simulink model "drive_cycle"  (R2019b)
settings: Solver=VariableStepAuto  StartTime=0.0  StopTime=1561  RelTol=1e-3
model workspace (MATLAB code in the model file):
  | ms = 135;
  | mf = 5;
  | mr = 10;
  | m = ms + (mf + mr);
  | a = 0.7;
  | b = 0.7;
  | Cd = 0.8;
  | Af = 1;
  | h_cg = 0.5;
  | kf = 10000;
  | kr = 15000;
  | cf = 5000;
  | cr = 5000;
  | I = 500;
  | kt = 175000;
  | GR = 6.5;
  | Pmax = 5500;
  | Tmax = 26;
libraries: autolibshared x4
(part 1 of 3)
settings Model: Creator=Barath Krishna S  LastModifiedBy=Barath Krishna S

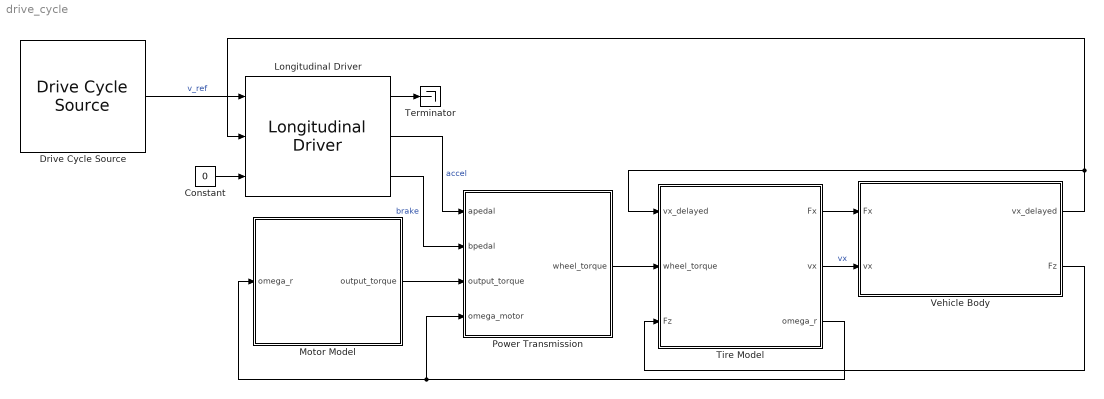
== system drive_cycle ==
  Constant : Constant  Value=0
  Drive Cycle Source : autolibshared/Drive Cycle Source  cycleVar=Workspace variable  wsVar=mycycle  fileVar=cycleFTP75.mat  tfinal="1560.636  seconds"  cycleRepeat=off  outAccPort=off  outGearPort=off  gearList=No gear data  t_wot1=5  xdot_woto=0  xdot_wot1=30  t_wot2=20  xdot_wot2=0  t_wotend=30  srcUnit=m/s  outUnit=m/s  srcAccUnit=m/s/s  outAccUnit=m/s^2  dt=0  aMode=1
      settings: SourceProductName=Powertrain Blockset  SourceProductBaseCode=PW
  Longitudinal Driver : autolibshared/Longitudinal Driver  cntrlType=PI  shftType=None  velUnits=m/s  gearOut=off  Kp=100  Ki=2.5  Kff=.05  Kg=.01  VehVelVec=[0 100]  KffVec=[.1 .1]  KpVec=[10 10]  KiVec=[5 5]  KgVec=[0 0]  m=1500  Kpt=3000  tau=.1  L=2  aR=200  bR=2.5  cR=.5  g=9.81  vnom=100  Kaw=.1  tauerr=.03  tauPt=2  GearInit=0  tShift=.1  pdlVec=[0.1 0.4 0.5 0.9]  upShftTbl=[-1 12.9375 26.4375 39.9375 51.18749999999999 62.4375 72.84375 83.25;-1 16.3125 29.8125 43.3125 54.5624 65.8125 76.78125 87.75;-1 19.6875 33.1875 46.68749999999999 57.9375 69.1875 80.71875 92.25;-1 33 52.5 77.25 100.5 138.75 161.875 185]  dwnShftTbl=[1 9.5625 23.0625 36.5625 47.8125 59.0625 68.90625 78.75;1 12.9375 26.4375 39.9375 51.18749999999999 62.4375 72.84375 83.25;1 16.3125 29.8125 43.3125 54.562499 65.8125 76.78125 87.75;1 19.6875 33.1875 46.68749999999999 57.9375 69.1875 80.71875 92.25]  tClutch=.5  tRev=.5  tPark=120  aMode=1  UpGearVec="[0  1  2  3  4  5  6  7]"  DownGearVec="[1  2  3  4  5  6  7  8]"
      settings: SourceProductName=Powertrain Blockset  SourceProductBaseCode=PW
  Motor Model : Subsystem
      mask Display: image('D:\Inter IIT\Plots & Images\BLDC-Motor.gif'); % Use "Edit Image" on toolstrip to change.
  Power Transmission : Subsystem
      mask Display: image('D:\Inter IIT\Plots & Images\electric-motor-shaft-500x500.jpg'); % Use "Edit Image" on toolstrip to change.
  Terminator : Terminator
  Tire Model : Subsystem
      mask Display: image('$imagefile'); % Use "Edit Image" on toolstrip to change.
  Vehicle Body : Subsystem
      mask Display: image('D:\Inter IIT\Plots & Images\Bicycle_model.jpg'); % Use "Edit Image" on toolstrip to change.
  wires:
  Tire Model/2(vx) -> Vehicle Body/2(vx)  "vx"
  Vehicle Body/2(Fz) -> Tire Model/3(Fz)
  Vehicle Body/1(vx_delayed) -> Longitudinal Driver/2, Tire Model/1(vx_delayed)
  Tire Model/1(Fx) -> Vehicle Body/1(Fx)
  Drive Cycle Source/1 -> Longitudinal Driver/1  "v_ref"
  Constant/1 -> Longitudinal Driver/3
  Longitudinal Driver/1 -> Terminator/1
  Longitudinal Driver/2 -> Power Transmission/1(apedal)  "accel"
  Longitudinal Driver/3 -> Power Transmission/2(bpedal)  "brake"
  Motor Model/1(output_torque) -> Power Transmission/3(output_torque)
  Power Transmission/1(wheel_torque) -> Tire Model/2(wheel_torque)
  Tire Model/3(omega_r) -> Power Transmission/4(omega_motor), Motor Model/1(omega_r)

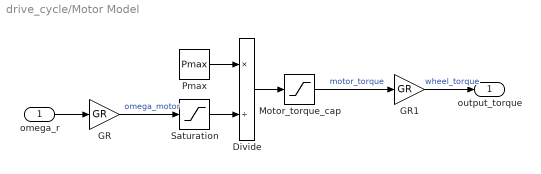
== system drive_cycle/Motor Model ==
  omega_r : Inport
  Divide : Product  Inputs=*/
  GR : Gain  Gain=GR
  GR1 : Gain  Gain=GR
  Motor_torque_cap : Saturate  UpperLimit=Tmax  LowerLimit=0
  Pmax : Constant  Value=Pmax
  Saturation : Saturate  UpperLimit=inf  LowerLimit=0.001
  output_torque : Outport
  wires:
  Pmax/1 -> Divide/1
  Saturation/1 -> Divide/2
  Divide/1 -> Motor_torque_cap/1
  omega_r/1 -> GR/1
  GR/1 -> Saturation/1  "omega_motor"
  Motor_torque_cap/1 -> GR1/1  "motor_torque"
  GR1/1 -> output_torque/1  "wheel_torque"

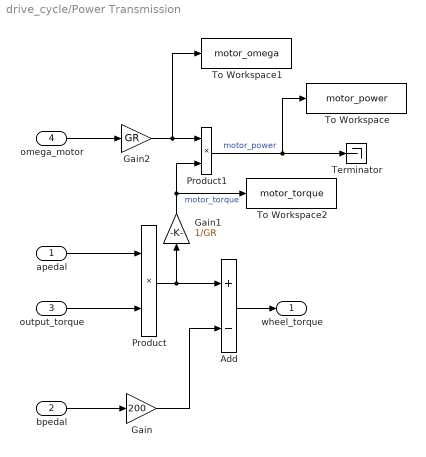
== system drive_cycle/Power Transmission ==
  apedal : Inport
  bpedal : Inport  Port=2
  output_torque : Inport  Port=3
  omega_motor : Inport  Port=4
  Add : Sum  Inputs=+-
  Gain : Gain  Gain=200
  Gain1 : Gain  Gain=1/GR
  Gain2 : Gain  Gain=GR
  Product : Product
  Product1 : Product
  Terminator : Terminator
  To Workspace : ToWorkspace  VariableName=motor_power  SampleTime=0.1
  To Workspace1 : ToWorkspace  VariableName=motor_omega  SampleTime=0.1
  To Workspace2 : ToWorkspace  VariableName=motor_torque  SampleTime=0.1
  wheel_torque : Outport
  wires:
  apedal/1 -> Product/1
  output_torque/1 -> Product/2
  bpedal/1 -> Gain/1
  Gain/1 -> Add/2
  Product/1 -> Add/1, Gain1/1
  Add/1 -> wheel_torque/1
  omega_motor/1 -> Gain2/1
  Product1/1 -> Terminator/1, To Workspace/1  "motor_power"
  Gain1/1 -> To Workspace2/1, Product1/2  "motor_torque"
  Gain2/1 -> To Workspace1/1, Product1/1
